simulink model "TEST"  (R2017b)
settings: Solver=FixedStepAuto  StartTime=0.0  StopTime=300  FixedStep=0.1  RelTol=1e-3
libraries: dspstat3 x1
settings Model: Creator=ghleila  LastModifiedBy=ghleila

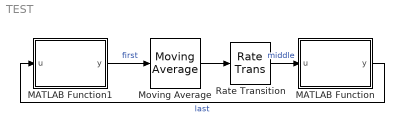
== system TEST ==
  MATLAB Function : MATLAB Function  TreatAsAtomicUnit=on
  MATLAB Function1 : MATLAB Function  TreatAsAtomicUnit=on
  Moving Average : dspstat3/Moving Average  Method=Sliding window  SpecifyWindowLength=on  WindowLength=4  ForgettingFactor=0.9  SimulateUsing=Code generation
  Rate Transition : RateTransition  OutPortSampleTime=20
  wires:
  MATLAB Function1/1(y) -> Moving Average/1  "first"
  Rate Transition/1 -> MATLAB Function/1(u)  "middle"
  Moving Average/1 -> Rate Transition/1
  MATLAB Function/1(y) -> MATLAB Function1/1(u)  "last"

== matlab function TEST/MATLAB Function1 ==
  data: u input; y output
function y = fcn(u)
%#codegen

if isempty(u)
    u=1;
end

y = 2*u*5;

== matlab function TEST/MATLAB Function ==
  data: u input; y output
function y = fcn(u)
%#codegen

y = 2*u;
